simulink model "testing"  (R2019b)
settings: Solver=ode4  StartTime=0.0  StopTime=t(end)  FixedStep=simIn.dt  RelTol=1e-3
values from neighbouring files (symbols this model uses):
  h = min(-kitepos(idx_nav,3)):1:max(-kitepos(idx_nav,3))    [Experimental_data.m]
  vw = 5.382*h.^0.1826    [Experimental_data.m]
undefined symbols (not defined in the file or in its folder): __PRM__SERIALIZED__DATA__, simIn, SubsystemReferenceBlock
settings Model: Creator=dylaneijkelhof  LastModifiedBy=dylaneijkelhof

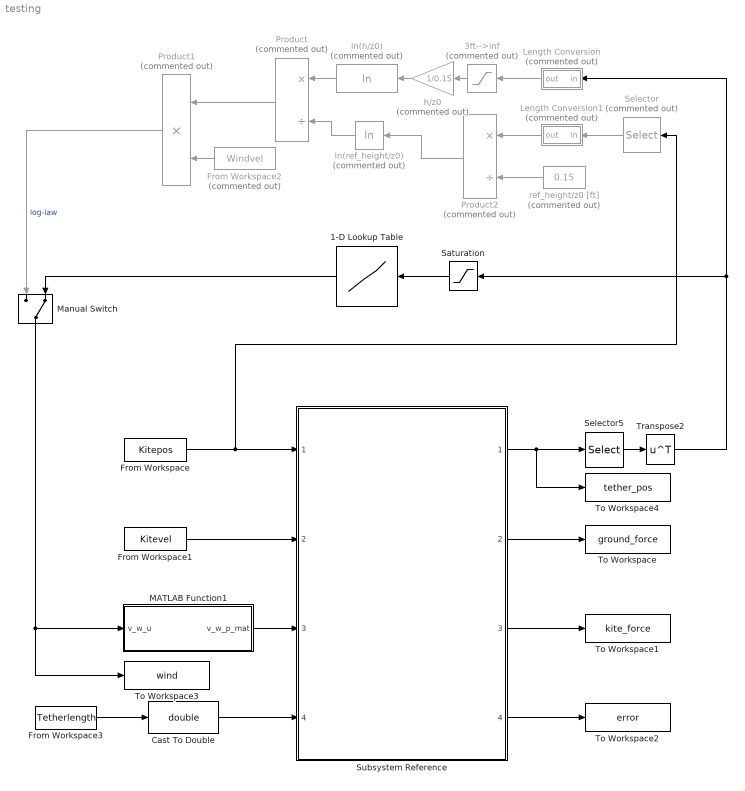
== system testing ==
  1-D Lookup Table : Lookup_n-D  NumberOfTableDimensions=1  BreakpointsForDimension1=h  Table=vw  InternalRulePriority=Speed  RndMeth=Simplest  InputSameDT=on
  3ft-->inf : Saturate  Commented=on  UpperLimit=inf  LowerLimit=3
  Cast To Double : DataTypeConversion  OutDataTypeStr=double  RndMeth=Nearest
  From Workspace : FromWorkspace  VariableName=Kitepos  SampleTime=simIn.dt  Interpolate=off  OutputAfterFinalValue=Holding final value
  From Workspace1 : FromWorkspace  VariableName=Kitevel  SampleTime=simIn.dt  Interpolate=off  OutputAfterFinalValue=Holding final value
  From Workspace2 : FromWorkspace  Commented=on  VariableName=Windvel  SampleTime=simIn.dt  Interpolate=off  OutputAfterFinalValue=Holding final value
  From Workspace3 : FromWorkspace  VariableName=Tetherlength  SampleTime=simIn.dt  Interpolate=off  OutputAfterFinalValue=Holding final value
  Length Conversion : Subsystem  Commented=on
  Length Conversion1 : Subsystem  Commented=on
  MATLAB Function1 : MATLAB Function  TreatAsAtomicUnit=on
  Manual Switch : ManualSwitch  CurrentSetting=0
  Product : Product  Commented=on  Inputs=*/  SaturateOnIntegerOverflow=on  InputSameDT=on  OutDataTypeStr=Inherit: Same as first input
  Product1 : Product  Commented=on  SaturateOnIntegerOverflow=on  InputSameDT=on  OutDataTypeStr=Inherit: Same as first input
  Product2 : Product  Commented=on  Inputs=*/  SaturateOnIntegerOverflow=on  InputSameDT=on  OutDataTypeStr=Inherit: Same as first input
  Saturation : Saturate  UpperLimit=max(h)  LowerLimit=min(h)
  Selector : Selector  Commented=on  InputPortWidth=3  IndexOptions=Index vector (dialog)  Indices=3  OutputSizes=1
  Selector5 : Selector  NumberOfDimensions=2  InputPortWidth=3  IndexOptions=Index vector (dialog),Select all  Indices=3,1  OutputSizes=1,1
  Subsystem Reference : Subsystem  BlockKeywords=__PRM__SERIALIZED__DATA__:SubsystemReferenceBlock  ReferencedSubsystem=Tether_dynamics_R2019B
  To Workspace : ToWorkspace  VariableName=ground_force  SaveFormat=Timeseries  SampleTime=-1
  To Workspace1 : ToWorkspace  VariableName=kite_force  SaveFormat=Timeseries  SampleTime=-1
  To Workspace2 : ToWorkspace  VariableName=error  SaveFormat=Timeseries  SampleTime=-1
  To Workspace3 : ToWorkspace  VariableName=wind  SaveFormat=Timeseries  SampleTime=-1
  To Workspace4 : ToWorkspace  VariableName=tether_pos  SaveFormat=Timeseries  SampleTime=-1
  Transpose2 : Math  Operator=transpose  SignedPower=off  SaturateOnIntegerOverflow=on
  h/z0 : Gain  Commented=on  Gain=1/0.15  SaturateOnIntegerOverflow=on  OutDataTypeStr=Inherit: Same as input  ParamDataTypeStr=Inherit: Same as input
  ln(h/z0) : Math  Commented=on  Operator=log  SaturateOnIntegerOverflow=on
  ln(ref_height/z0) : Math  Commented=on  Operator=log  SaturateOnIntegerOverflow=on
  ref_height/z0 [ft] : Constant  Commented=on  Value=0.15  OutDataTypeStr=Inherit: Inherit via back propagation
  wires:
  From Workspace/1 -> Selector/1, Subsystem Reference/1
  From Workspace1/1 -> Subsystem Reference/2
  From Workspace3/1 -> Cast To Double/1
  Subsystem Reference/3 -> To Workspace1/1
  Subsystem Reference/2 -> To Workspace/1
  Subsystem Reference/1 -> To Workspace4/1, Selector5/1
  Subsystem Reference/4 -> To Workspace2/1
  Cast To Double/1 -> Subsystem Reference/4
  Selector5/1 -> Transpose2/1
  MATLAB Function1/1(v_w_p_mat) -> Subsystem Reference/3
  h/z0/1 -> ln(h/z0)/1
  ln(ref_height/z0)/1 -> Product/2
  Length Conversion/1(out) -> 3ft-->inf/1
  Transpose2/1 -> Length Conversion/1(in), Saturation/1
  ln(h/z0)/1 -> Product/1
  ref_height/z0 [ft]/1 -> Product2/2
  3ft-->inf/1 -> h/z0/1
  Product1/1 -> Manual Switch/1  "log-law"
  Product/1 -> Product1/1
  From Workspace2/1 -> Product1/2
  Product2/1 -> ln(ref_height/z0)/1
  Length Conversion1/1(out) -> Product2/1
  Selector/1 -> Length Conversion1/1(in)
  Saturation/1 -> 1-D Lookup Table/1
  1-D Lookup Table/1 -> Manual Switch/2
  Manual Switch/1 -> MATLAB Function1/1(v_w_u), To Workspace3/1

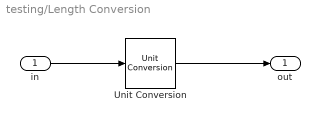
== system testing/Length Conversion ==
  in : Inport  Unit=m
  Unit Conversion : UnitConversion
  out : Outport  Unit=ft  VectorParamsAs1DForOutWhenUnconnected=off
  wires:
  in/1 -> Unit Conversion/1
  Unit Conversion/1 -> out/1

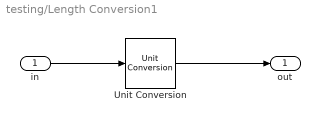
== system testing/Length Conversion1 ==
  in : Inport  Unit=m
  Unit Conversion : UnitConversion
  out : Outport  Unit=ft  VectorParamsAs1DForOutWhenUnconnected=off
  wires:
  in/1 -> Unit Conversion/1
  Unit Conversion/1 -> out/1

== matlab function testing/MATLAB Function1 ==
  data: v_w_u input; v_w_p_mat output
% Copyright 2021 Delft University of Technology
%
% Licensed under the Apache License, Version 2.0 (the "License");
% you may not use this file except in compliance with the License.
% You may obtain a copy of the License at
%
%      http://www.apache.org/licenses/LICENSE-2.0
%
% Unless required by applicable law or agreed to in writing, software
% distributed under the License is distributed on an "AS IS" BASIS,
% WITHOUT WARRANTIES OR CONDITIONS OF ANY KIND, either express or implied.
% See the License for the specific language governing permissions and
% limitations under the License.

function v_w_p_mat = fcn(v_w_u)

v_w_p_mat = zeros( 3, length( v_w_u) );
v_w_p_mat(1,:) = v_w_u';
